simulink model "mip_balance"  (R2017b)
settings: Solver=FixedStepDiscrete  StartTime=0.0  StopTime=inf  RelTol=1e-3  EnableMultiTasking=on
undefined symbols (not defined in the file): DiscIntNeverNeededParam
libraries: beaglebonebluelib x6, simulink_extras x1
settings Model: FPTRunName=Active  SimulationMode=external  ExtModeTrigDuration=2  Creator=The MathWorks, Inc.  LastModifiedBy=pthb3
settings SolverCC: PositivePriorityOrder=on
settings DataIOCC: LimitDataPoints=on  SaveFormat=Array
settings OptimizationCC: ExpressionDepthLimit=2147483647  LifeSpan=Inf  MaxStackSize=64
settings DebuggingCC: UnderspecifiedInitializationDetection=Classic  MergeDetectMultiDrivingBlocksExec=none  FcnCallInpInsideContextMsg=warning  AllowSymbolicDim=off  StateNameClashWarn=warning  SFUnexpectedBacktrackingDiag=warning  SFNoUnconditionalDefaultTransitionDiag=warning  SFExecutionAtInitializationDiag=none
settings HardwareCC: ProdBitPerPointer=32  ProdBitPerSizeT=32  ProdBitPerPtrDiffT=32  ProdLargestAtomicInteger=Long  ProdLargestAtomicFloat=Double  ProdWordSize=32  ProdHWDeviceType=ARM Compatible->ARM Cortex  UseEmbeddedCoderFeatures=off
settings ModelReferenceCC: PropagateSignalLabelsOutOfModel=off
settings RTWCC: SystemTargetFile=ert.tlc  HardwareBoard=BeagleBone Blue  TemplateMakefile=ert_default_tmf  RTWVerbose=off  Toolchain=GNU GCC BeagleBone Blue
settings CodeAppCC: StateflowObjectComments=on
settings ERTTargetCC: MultiwordLength=2048  ERTCustomFileBanners=off  SupportContinuousTime=on  SupportNonInlinedSFcns=on  RemoveResetFunc=off  SupportVariableSizeSignals=on  ModelStepFunctionPrototypeControlCompliant=off  ConvertIfToSwitch=off  SuppressUnreachableDefaultCases=off
settings ConfigComp: CovMetricSettings=dw  CovHtmlReporting=on  CovSaveCumulativeToWorkspaceVar=on  CovSaveSingleToWorkspaceVar=on  CovExternalEMLEnable=off  CovSFcnEnable=off

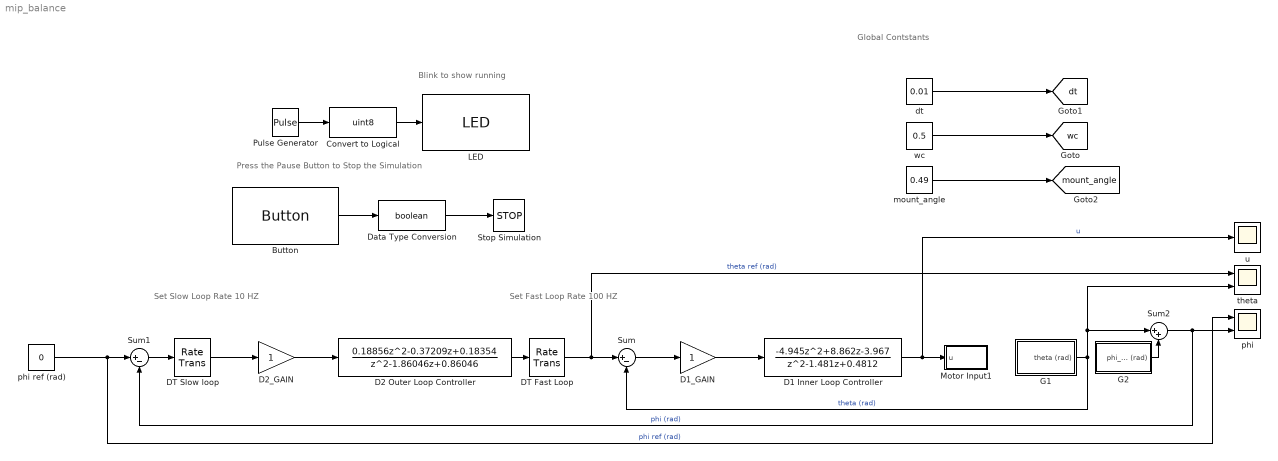
== system mip_balance ==
  note: Global Contstants
  note: Press the Pause Button to Stop the Simulation
  note: Blink to show running
  note: Set Fast Loop Rate
      | 100 HZ
  note: Set Slow Loop Rate
      | 10 HZ
  Button : beaglebonebluelib/Button  Button=Pause  SampleTime=0.1  SimulateUsing=Code generation
      settings: SourceProductName=Simulink Coder Support Package for BeagleBone Blue Hardware
  Convert to Logical : DataTypeConversion  OutDataTypeStr=uint8
  D1 Inner Loop Controller : DiscreteTransferFcn  Numerator=[-4.945, 8.862, -3.967]  Denominator=[1.000, -1.481, 0.4812]
  D1_GAIN : Gain
  D2 Outer Loop Controller : DiscreteTransferFcn  Numerator="[0.18856,  -0.37209,  0.18354]"  Denominator="[1.00000,  -1.86046,   0.86046]"
  D2_GAIN : Gain
  DT Fast Loop : RateTransition  OutPortSampleTimeOpt=Multiple of input port sample time  OutPortSampleTimeMultiple=0.1  OutPortSampleTime=0.05
  DT Slow loop : RateTransition  OutPortSampleTime=0.1
  Data Type Conversion : DataTypeConversion  OutDataTypeStr=boolean
  G1 : Subsystem
  G2 : Subsystem
  LED : beaglebonebluelib/LED  LED=Green
      settings: SourceProductName=Simulink Coder Support Package for BeagleBone Blue Hardware
  Motor Input1 : Subsystem  TreatAsAtomicUnit=on
  Pulse Generator : DiscretePulseGenerator  Period=10  PulseWidth=5  SampleTime=0.1
  Stop Simulation : Stop
  Sum : Sum  Inputs=|+-
  Sum1 : Sum  Inputs=|+-
  Sum2 : Sum  Inputs=|++
  dt : Constant  Value=0.01
  mount_angle : Constant  Value=0.49
  phi : Scope  NumInputPorts=2
  phi ref (rad) : Constant  Value=0
  theta : Scope  NumInputPorts=2
  u : Scope
  wc : Constant  Value=0.5
  tag scope: dt=global, mount_angle=global, wc=global
  wires:
  Convert to Logical/1 -> LED/1
  Pulse Generator/1 -> Convert to Logical/1
  Data Type Conversion/1 -> Stop Simulation/1
  Button/1 -> Data Type Conversion/1
  DT Slow loop/1 -> D2_GAIN/1
  wc/1 -> [wc]
  G1/1(theta (rad)) -> theta/2, Sum2/1, Sum/2  "theta (rad)"
  G2/1(phi_enc (rad)) -> Sum2/2
  D2_GAIN/1 -> D2 Outer Loop Controller/1
  Sum/1 -> D1_GAIN/1
  Sum2/1 -> Sum1/2, phi/2  "phi (rad)"
  phi ref (rad)/1 -> phi/1, Sum1/1  "phi ref (rad)"
  dt/1 -> [dt]
  D1 Inner Loop Controller/1 -> Motor Input1/1(u), u/1  "u"
  D1_GAIN/1 -> D1 Inner Loop Controller/1
  D2 Outer Loop Controller/1 -> DT Fast Loop/1
  Sum1/1 -> DT Slow loop/1
  DT Fast Loop/1 -> theta/1, Sum/1  "theta ref (rad)"
  mount_angle/1 -> [mount_angle]

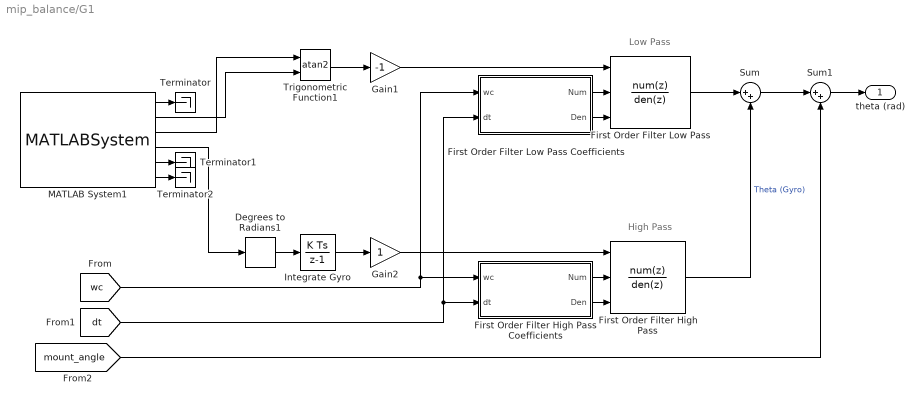
== system mip_balance/G1 ==
  note: High Pass
  note: Low Pass
  Degrees to Radians1 : simulink_extras/Transformations/Degrees to Radians
  First Order Filter High Pass : DiscreteTransferFcn  NumeratorSource=Input port  DenominatorSource=Input port  Denominator=[1]  a0EqualsOne=on
      settings: InputPortMap=u0,p1,p3
  First Order Filter High Pass Coefficients : MATLAB Function  TreatAsAtomicUnit=on
  First Order Filter Low Pass : DiscreteTransferFcn  NumeratorSource=Input port  DenominatorSource=Input port  Denominator=[1]  a0EqualsOne=on
      settings: InputPortMap=u0,p1,p3
  First Order Filter Low Pass Coefficients : MATLAB Function  TreatAsAtomicUnit=on
  Gain1 : Gain  Gain=-1
  Gain2 : Gain
  Integrate Gyro : DiscreteIntegrator  InitialConditionSetting=State (most efficient)  SampleTime=-1  ICPrevOutput=DiscIntNeverNeededParam  ICPrevScaledInput=DiscIntNeverNeededParam
  MATLAB System1 : MATLABSystem  System=beagleboneblue.fccr_bbblueIMU  SampleTime=0.01
      mask Type: beagleboneblue.fccr_bbblueIMU
      mask Display:
      | color('white');
      | plot([100,100,100,100]*1,[100,100,100,100]*1);
      | plot([100,100,100,100]*0,[100,100,100,100]*0);
      | color('blue');
      | text(100, 92, ' BB BLUE ', 'horizontalAlignment', 'right');
      | color('black');
      | text(52,52,' IMU','horizontalAlignment','center');
      | color('black');
  Sum : Sum  Inputs=|++
  Sum1 : Sum  Inputs=|++
  Terminator : Terminator
  Terminator1 : Terminator
  Terminator2 : Terminator
  Trigonometric Function1 : Trigonometry  Operator=atan2
  theta (rad) : Outport
  wires:
  First Order Filter Low Pass Coefficients/1(Num) -> First Order Filter Low Pass/2
  Gain2/1 -> First Order Filter High Pass/1
  First Order Filter Low Pass Coefficients/2(Den) -> First Order Filter Low Pass/3
  MATLAB System1/4 -> Degrees to Radians1/1
  Trigonometric Function1/1 -> Gain1/1
  [wc] -> First Order Filter Low Pass Coefficients/1(wc), First Order Filter High Pass Coefficients/1(wc)
  [dt] -> First Order Filter Low Pass Coefficients/2(dt), First Order Filter High Pass Coefficients/2(dt)
  First Order Filter High Pass Coefficients/2(Den) -> First Order Filter High Pass/3
  First Order Filter Low Pass/1 -> Sum/1
  Gain1/1 -> First Order Filter Low Pass/1
  Integrate Gyro/1 -> Gain2/1
  First Order Filter High Pass/1 -> Sum/2  "Theta (Gyro)"
  Degrees to Radians1/1 -> Integrate Gyro/1
  Sum/1 -> Sum1/1
  MATLAB System1/2 -> Trigonometric Function1/2
  First Order Filter High Pass Coefficients/1(Num) -> First Order Filter High Pass/2
  MATLAB System1/3 -> Trigonometric Function1/1
  Sum1/1 -> theta (rad)/1
  [mount_angle] -> Sum1/2
  MATLAB System1/1 -> Terminator/1
  MATLAB System1/5 -> Terminator1/1
  MATLAB System1/6 -> Terminator2/1

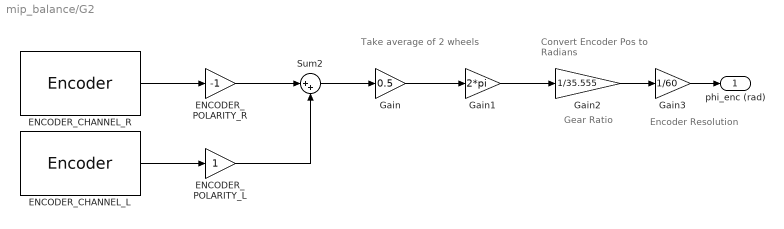
== system mip_balance/G2 ==
  note: Encoder
      | Resolution
  note: Gear Ratio
  note: Convert Encoder Pos
      | to Radians
  note: Take average
      | of 2 wheels
  ENCODER_CHANNEL_L : beaglebonebluelib/Encoder  Channel=3  Mode=No reset  SampleTime=0.01  SimulateUsing=Code generation
      settings: SourceProductName=Simulink Coder Support Package for BeagleBone Blue Hardware
  ENCODER_CHANNEL_R : beaglebonebluelib/Encoder  Channel=2  Mode=No reset  SampleTime=0.01  SimulateUsing=Code generation
      settings: SourceProductName=Simulink Coder Support Package for BeagleBone Blue Hardware
  ENCODER_POLARITY_L : Gain
  ENCODER_POLARITY_R : Gain  Gain=-1
  Gain : Gain  Gain=0.5  OutDataTypeStr=double
  Gain1 : Gain  Gain=2*pi
  Gain2 : Gain  Gain=1/35.555
  Gain3 : Gain  Gain=1/60
  Sum2 : Sum  Inputs=|++
  phi_enc (rad) : Outport
  wires:
  ENCODER_POLARITY_R/1 -> Sum2/1
  ENCODER_POLARITY_L/1 -> Sum2/2
  ENCODER_CHANNEL_L/1 -> ENCODER_POLARITY_L/1
  ENCODER_CHANNEL_R/1 -> ENCODER_POLARITY_R/1
  Sum2/1 -> Gain/1
  Gain/1 -> Gain1/1
  Gain1/1 -> Gain2/1
  Gain2/1 -> Gain3/1
  Gain3/1 -> phi_enc (rad)/1

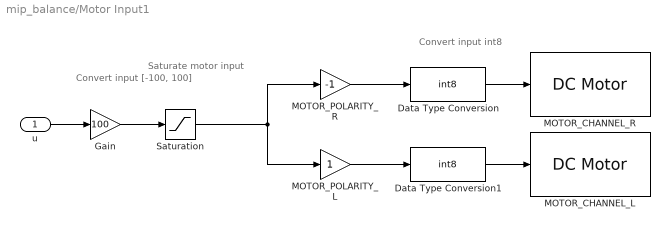
== system mip_balance/Motor Input1 ==
  note: Convert input
      | [-100, 100]
  note: Convert input
      | int8
  note: Saturate motor
      | input
  u : Inport
  Data Type Conversion : DataTypeConversion  OutDataTypeStr=int8  SaturateOnIntegerOverflow=on  RndMeth=Zero
  Data Type Conversion1 : DataTypeConversion  OutDataTypeStr=int8  SaturateOnIntegerOverflow=on  RndMeth=Zero
  Gain : Gain  Gain=100
  MOTOR_CHANNEL_L : beaglebonebluelib/DC Motor  index=3  stopaction=Free Spin  SimulateUsing=Code generation
      settings: SourceProductName=Simulink Coder Support Package for BeagleBone Blue Hardware
  MOTOR_CHANNEL_R : beaglebonebluelib/DC Motor  index=2  stopaction=Free Spin  SimulateUsing=Code generation
      settings: SourceProductName=Simulink Coder Support Package for BeagleBone Blue Hardware
  MOTOR_POLARITY_L : Gain
  MOTOR_POLARITY_R : Gain  Gain=-1
  Saturation : Saturate  UpperLimit=100  LowerLimit=-100  RndMeth=Zero
  wires:
  MOTOR_POLARITY_R/1 -> Data Type Conversion/1
  MOTOR_POLARITY_L/1 -> Data Type Conversion1/1
  u/1 -> Gain/1
  Gain/1 -> Saturation/1
  Saturation/1 -> MOTOR_POLARITY_R/1, MOTOR_POLARITY_L/1
  Data Type Conversion/1 -> MOTOR_CHANNEL_R/1
  Data Type Conversion1/1 -> MOTOR_CHANNEL_L/1

== matlab function mip_balance/G1/First Order Filter High Pass Coefficients ==
  data: wc input; Num output; dt input; Den output
function [Num, Den] = first_order_hp(wc,dt)
%#codegen
Num = [1 -1];
Den = [1 (wc*dt - 1)];

== matlab function mip_balance/G1/First Order Filter Low Pass Coefficients ==
  data: wc input; Num output; dt input; Den output
function [Num, Den] = first_order_lp(wc,dt)
%#codegen
Num = [0 wc*dt];
Den = [1 (wc*dt - 1)];
